simulink model "Pend_MSAM_PP_noObserver"  (Simulink 7.9)
settings: Solver=ode45  StartTime=0.0  StopTime=time_span  RelTol=1e-3
values from neighbouring files (symbols this model uses):
  outstr = sim_model    [RunCtrlModel.m]    (also in RunPertModels_sym.m = GetEqnStr_sym(model_eqns(j),p.allvars,'eqn'))
  samp_time = p.simulation.samp_time    [RunCtrlModel.m]    (also in RunPertModels_sym.m)
undefined symbols (not defined in the file or in its folder): p
libraries: dspsrcs4 x1
settings Model: Creator=KushalSahare  LastModifiedBy=Kourosh Danai
settings GRTTargetCC: CombineOutputUpdateFcns=off  GRTInterface=on

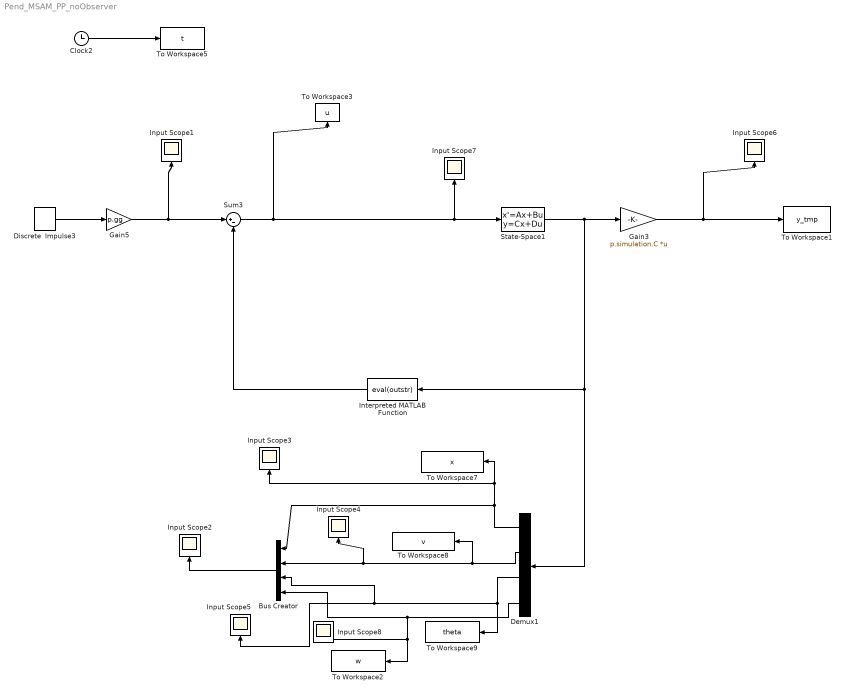
== system Pend_MSAM_PP_noObserver ==
  Bus Creator : BusCreator
  Clock2 : Clock
  Demux1 : Demux
  Discrete  Impulse3 : dspsrcs4/Discrete  Impulse  Delay=0  SampleTime=1  FrameSample=1  dataType=double  isSigned=on  wordLen=16  udDataType=sfix(16)  fracBitsMode=Best precision  numFracBits=15  OutDataTypeStr=double  LastOutDataTypeStr=double
  Gain3 : Gain  Gain=p.simulation.C  Multiplication=Matrix(K*u) (u vector)
  Gain5 : Gain  Gain=p.gg
  Input Scope{1..8} (8 alike) : Scope
      Input Scope3 settings: SaveName=ScopeData2
      Input Scope4 settings: SaveName=ScopeData3
      Input Scope5 settings: SaveName=ScopeData4
      Input Scope6 settings: SaveName=ScopeData5
      Input Scope7 settings: SaveName=ScopeData6
      Input Scope8 settings: SaveName=ScopeData7
  Interpreted MATLAB Function : MATLABFcn  MATLABFcn=eval(outstr)
  State-Space1 : StateSpace  A=p.simulation.A  B=p.simulation.B  C=[1,0,0,0;0,1,0,0;0,0,1,0;0,0,0,1]  D=[0;0;0;0]  X0=[0;0;0;0]
  Sum3 : Sum  Inputs=|+-
  To Workspace1 : ToWorkspace  VariableName=y_tmp  SampleTime=samp_time
  To Workspace2 : ToWorkspace  VariableName=w  SampleTime=samp_time
  To Workspace3 : ToWorkspace  VariableName=u  SampleTime=samp_time
  To Workspace5 : ToWorkspace  VariableName=t  SampleTime=samp_time
  To Workspace7 : ToWorkspace  VariableName=x  SampleTime=samp_time
  To Workspace8 : ToWorkspace  VariableName=v  SampleTime=samp_time
  To Workspace9 : ToWorkspace  VariableName=theta  SampleTime=samp_time
  wires:
  Clock2/1 -> To Workspace5/1
  Discrete  Impulse3/1 -> Gain5/1
  Sum3/1 -> To Workspace3/1, State-Space1/1, Input Scope7/1
  Gain5/1 -> Input Scope1/1, Sum3/1
  Gain3/1 -> Input Scope6/1, To Workspace1/1
  State-Space1/1 -> Gain3/1, Demux1/1, Interpreted MATLAB Function/1
  Demux1/1 -> Bus Creator/1, To Workspace7/1, Input Scope3/1
  Demux1/2 -> To Workspace8/1, Bus Creator/2, Input Scope4/1
  Demux1/3 -> To Workspace9/1, Input Scope5/1, Bus Creator/3
  Interpreted MATLAB Function/1 -> Sum3/2
  Bus Creator/1 -> Input Scope2/1
  Demux1/4 -> Bus Creator/4, To Workspace2/1, Input Scope8/1
